simulink model "VIENNA_"  (R2021a)
settings: Solver=ode45  StartTime=0.0  StopTime=0.45  RelTol=1e-3  EnableMultiTasking=on
libraries: spsDiodeLib x6, spsMosfetLib x6, spsSeriesRLCBranchLib x6, spsVoltageMeasurementLib x3, spsCurrentMeasurementLib x1, spsDCMachineLib x1, spsDCVoltageSourceLib x1, spsMeanLib x1, spsPower3phInstantaneousLib x1, slpidlib x1, spsThreePhaseVIMeasurementLib x1, spsThreePhaseSourceLib x1
settings Model: Creator=Zhaoxuqiang  LastModifiedBy=Saghana
settings SolverCC: AlgebraicLoopSolver=TrustRegion
settings DataIOCC: LimitDataPoints=on  SaveFormat=Array  ReturnWorkspaceOutputs=off
settings OptimizationCC: LifeSpan=inf
settings DebuggingCC: SolverPrmCheckMsg=warning  SFUnexpectedBacktrackingDiag=warning  SFNoUnconditionalDefaultTransitionDiag=warning  SFExecutionAtInitializationDiag=none  SFMachineParentedDataDiag=warning  ArithmeticOperatorsInVariantConditions=warning
settings HardwareCC: ProdBitPerPointer=32  ProdBitPerSizeT=32  ProdBitPerPtrDiffT=32  ProdLargestAtomicFloat=None  ProdIntDivRoundTo=Undefined  ProdEndianess=Unspecified  ProdWordSize=32  ProdHWDeviceType=32-bit Generic
settings ModelReferenceCC: PropagateSignalLabelsOutOfModel=off
settings SFSimCC: SimUseLocalCustomCode=off  CustomCodeUndefinedFunction=UseInterfaceOnly
settings RTWCC: RTWUseLocalCustomCode=off
settings CodeAppCC: StateflowObjectComments=on
settings GRTTargetCC: TargetLangStandard=C89/C90 (ANSI)
settings ConfigComp: CovMetricSettings=dw  CovSaveCumulativeToWorkspaceVar=on  CovSaveSingleToWorkspaceVar=on  CovExternalEMLEnable=off  CovSFcnEnable=off
settings SimscapeCC: SimscapeNormalizeSystem=off

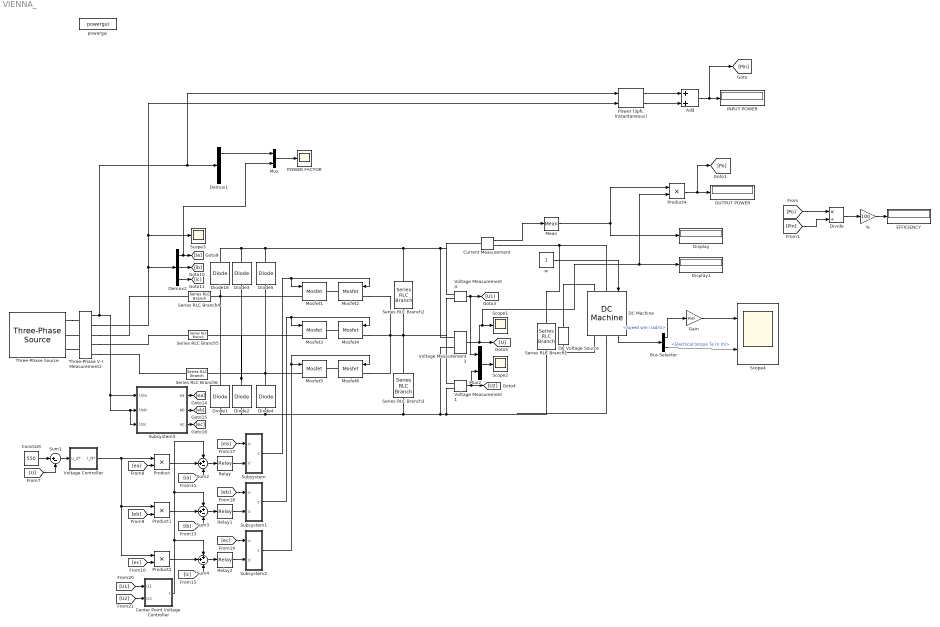
== system VIENNA_ ==
  % : Gain  Gain=100
  Add : Sum
  Bus Selector : BusSelector  OutputSignals=Speed wm (rad/s),Electrical torque Te (n m)
  Center Point Voltage Controller : Subsystem
  Constant : Constant  Value=550
  Current Measurement : spsCurrentMeasurementLib/Current Measurement  PhasorSimulation=off  OutputType=Complex  PSBequivalent=0
  DC Machine : spsDCMachineLib/DC Machine  PresetModel=03: 5HP 500V 1750RPM Field:300V  MechanicalLoad=Torque TL  FieldType=Wound  ShowDetailedParameters=on  MeasurementBus=off  RLa=[11.2 0.1215]  RLf=[281.2 156]  Laf=1.976  MachineConstant=Torque constant (N.m/A)  Ke=1.8  Kt=1.8  J=0.02215  Bm=0.002953  Tf=0.5161  w0=1  Ifinit=1.06685632871799  TsPowergui=0  TsBlock=-1
  DC Voltage Source : spsDCVoltageSourceLib/DC Voltage Source  Amplitude=300  Measurements=None
  Demux1 : Demux  Outputs=3
  Demux2 : Demux  Outputs=3
  Diode{1..5,18} (6 alike) : spsDiodeLib/Diode  Ron=0.001  Lon=0  Vf=0.8  IC=0  UseSnubber=off  Rs=500  Cs=250e-9  Measurements=off
  Display : Display
  Display1 : Display
  Divide : Product  Inputs=*/
  EFFICIENCY : Display
  Gain : Gain  Gain=30/pi
  INPUT POWER : Display
  Mean : spsMeanLib/Mean  Freq=60  Vinit=0  Ts=0
  Mosfet{1..6} (6 alike) : spsMosfetLib/Mosfet  Ron=0.1  Lon=0  Rd=0.01  Vfd=0  IC=0  Rs=1e5  Cs=inf  Measurements=off
  Mux : Mux  Inputs=2
  Mux2 : Mux  Inputs=2
  OUTPUT POWER : Display
  POWER FACTOR : Scope
  "Power (3ph, Instantaneous)" : spsPower3phInstantaneousLib/Power (3ph, Instantaneous)
  Product : Product  RndMeth=Zero
  Product1 : Product  RndMeth=Zero
  Product2 : Product  RndMeth=Zero
  Product4 : Product
  Relay : Relay  OnSwitchValue=1  OffSwitchValue=-1
  Relay1 : Relay  OnSwitchValue=1  OffSwitchValue=-1
  Relay2 : Relay  OnSwitchValue=1  OffSwitchValue=-1
  Scope1 : Scope
  Scope2 : Scope
  Scope3 : Scope
  Scope4 : Scope  NumInputPorts=2
  Series RLC Branch1 : spsSeriesRLCBranchLib/Series RLC Branch  LConnTagsString=__new0  RConnTagsString=__new0  BranchType=R  Resistance=50  Inductance=1e-3  SetiL0=off  InitialCurrent=0  Capacitance=4000e-6  Setx0=on  InitialVoltage=200  Measurements=None
  Series RLC Branch2 : spsSeriesRLCBranchLib/Series RLC Branch  LConnTagsString=__new0  RConnTagsString=__new0  BranchType=C  Resistance=0.001  Inductance=1e-3  SetiL0=off  InitialCurrent=0  Capacitance=4000e-6  Setx0=on  InitialVoltage=200  Measurements=None
  Series RLC Branch3 : spsSeriesRLCBranchLib/Series RLC Branch  LConnTagsString=__new0  RConnTagsString=__new0  BranchType=C  Resistance=0.002  Inductance=1e-3  SetiL0=off  InitialCurrent=0  Capacitance=4000e-6  Setx0=on  InitialVoltage=400  Measurements=None
  Series RLC Branch4 : spsSeriesRLCBranchLib/Series RLC Branch  LConnTagsString=__new0  RConnTagsString=__new0  BranchType=L  Resistance=1  Inductance=0.3e-3  SetiL0=off  InitialCurrent=0  Capacitance=1e-6  Setx0=off  InitialVoltage=0  Measurements=None
  Series RLC Branch5 : spsSeriesRLCBranchLib/Series RLC Branch  LConnTagsString=__new0  RConnTagsString=__new0  BranchType=L  Resistance=1  Inductance=0.3e-3  SetiL0=off  InitialCurrent=0  Capacitance=1e-6  Setx0=off  InitialVoltage=0  Measurements=None
  Series RLC Branch6 : spsSeriesRLCBranchLib/Series RLC Branch  LConnTagsString=__new0  RConnTagsString=__new0  BranchType=L  Resistance=1  Inductance=0.3e-3  SetiL0=off  InitialCurrent=0  Capacitance=1e-6  Setx0=off  InitialVoltage=0  Measurements=None
  Subsystem : Subsystem
  Subsystem1 : Subsystem
  Subsystem2 : Subsystem
  Subsystem3 : Subsystem
      mask Display: disp('PLL');
  Sum1 : Sum  Inputs=|+-
  Sum2 : Sum  Inputs=++-
  Sum3 : Sum  Inputs=++-
  Sum4 : Sum  Inputs=++-
  Three-Phase V-I Measurement2 : spsThreePhaseVIMeasurementLib/Three-Phase V-I Measurement  VoltageMeasurement=phase-to-ground  SetLabelV=off  LabelV=Uabc  Vpu=off  VpuLL=off  CurrentMeasurement=yes  SetLabelI=off  LabelI=Iabc  Ipu=off  Pbase=100e6  Vbase=500e3  OutputType=Complex  PhasorSimulation=off  PSBequivalent=0
  Three-Phase Source : spsThreePhaseSourceLib/Three-Phase Source  InternalConnection=Yg  VoltagePhases=off  Voltage=380  PhaseAngle=0  Voltage_phases=[25e3 25e3 25e3]/sqrt(3)  PhaseAngles_phases=[0 -120 +120]  Frequency=50  NonIdealSource=on  SpecifyImpedance=off  Resistance=0.000001  Inductance=0  ShortCircuitLevel=100e6  BaseVoltage=25e3  XRratio=7  BusType=swing  Pref=0  Qref=0  Prefabc=[10e3, 10e3, 10e3]  Qrefabc=[0, 0, 0]  Qmin=-inf  Qmax=inf
  Voltage Controller : Subsystem
      mask Display: disp('PI');
  Voltage Measurement1 : spsVoltageMeasurementLib/Voltage Measurement  PhasorSimulation=off  OutputType=Complex  PSBequivalent=0
  Voltage Measurement3 : spsVoltageMeasurementLib/Voltage Measurement  PhasorSimulation=off  OutputType=Complex  PSBequivalent=0
  Voltage Measurement4 : spsVoltageMeasurementLib/Voltage Measurement  PhasorSimulation=off  OutputType=Complex  PSBequivalent=0
  powergui : spspowerguiLib/powergui  SimulationMode=Continuous  SampleTime=1e-6  frequency=60  Iterations=50  frequencyindice=50  Pbase=100e6  ErrMax=1e-4  UnitsV=kV  UnitsW=MW  buscounter=0  FunctionMessages=off  echomessages=off  EnableUseOfTLC=off  CurrentSourceSwitches=on  DisableSnubberDevices=off  DisableRonSwitches=off  DisableVfSwitches=off  DisplayEquations=off  AutomaticDiscreteSolvers=off  SolverType=Tustin/Backward Euler (TBE)  Interpol=off  ExternalGateDelay=off  methode=off  Ts=0  x0status=blocks  SPID=off  SwTol=0  HookPort=off  NonlinearTolerance=1e-4  nMaxIteration=100  ContinueOnMaxIteration=off  RestoreLinks=warning  ResistiveCurrentMeasurement=off  Frange=[0:2:500]  Ylog=off  Xlog=on  ShowGrid=off  save=off  variable=ZData  structure=Iabc  ZoomFFT=off  StartTime=0.3  cycles=10  DisplayStyle=1  fundamental=50  FreqAxis=on  MaxFrequency=2500  frequencyindicesteady=1  RmsSteady=1  display=off
  w : Constant
  wires:
  Voltage Measurement3/1 -> Product4/2, Display1/1, Scope1/1, [U]
  Voltage Measurement1/1 -> Mux2/2, [U2]
  Voltage Measurement4/1 -> Mux2/1, [U1]
  Constant/1 -> Sum1/1
  Sum1/1 -> Voltage Controller/1(u_d*)
  [U] -> Sum1/2
  [ea] -> Product/2
  [eb] -> Product1/2
  Voltage Controller/1(I_N*) -> Product2/1, Product1/1, Product/1
  [ec] -> Product2/2
  Product/1 -> Sum2/2
  Demux2/2 -> [ib]
  Demux2/1 -> Mux/2, [ia]
  Demux2/3 -> [ic]
  [ia] -> Sum2/3
  Product1/1 -> Sum3/2
  [ib] -> Sum3/3
  Product2/1 -> Sum4/2
  [ic] -> Sum4/3
  Center Point Voltage Controller/1(I) -> Sum4/1, Sum3/1, Sum2/1
  Relay/1 -> Subsystem/2(s')
  [ea] -> Subsystem/1(u)
  Sum2/1 -> Relay/1
  Relay1/1 -> Subsystem1/2(s')
  [eb] -> Subsystem1/1(u)
  Sum3/1 -> Relay1/1
  Relay2/1 -> Subsystem2/2(s')
  [ec] -> Subsystem2/1(u)
  Sum4/1 -> Relay2/1
  [U1] -> Center Point Voltage Controller/1(U1)
  [U2] -> Center Point Voltage Controller/2(U2)
  Subsystem/1(s) -> Mosfet2/1, Mosfet1/1
  Subsystem1/1(s) -> Mosfet4/1, Mosfet3/1
  Subsystem2/1(s) -> Mosfet5/1, Mosfet6/1
  Three-Phase V-I Measurement2/1 -> "Power (3ph, Instantaneous)"/1, Demux1/1, Subsystem3/1(Uoa), Subsystem3/3(Uoc), Subsystem3/2(Uob)
  Subsystem3/1(ea) -> [ea]
  Subsystem3/2(eb) -> [eb]
  Subsystem3/3(ec) -> [ec]
  Mux2/1 -> Scope2/1
  w/1 -> DC Machine/1
  DC Machine/1 -> Bus Selector/1
  Bus Selector/1 -> Gain/1  "<Speed wm (rad/s)>"
  Bus Selector/2 -> Scope4/2  "<Electrical torque Te (n m)>"
  Mux/1 -> POWER FACTOR/1
  Current Measurement/1 -> Mean/1
  Demux1/1 -> Mux/1
  Gain/1 -> Scope4/1
  Product4/1 -> [Po], OUTPUT POWER/1
  "Power (3ph, Instantaneous)"/1 -> Add/1
  "Power (3ph, Instantaneous)"/2 -> Add/2
  Add/1 -> INPUT POWER/1, [Pin]
  [Po] -> Divide/1
  [Pin] -> Divide/2
  Divide/1 -> %/1
  %/1 -> EFFICIENCY/1
  Mean/1 -> Display/1, Product4/1
  Three-Phase V-I Measurement2/2 -> "Power (3ph, Instantaneous)"/2, Scope3/1, Demux2/1
  connections:
  Three-Phase V-I Measurement2/RConn3 -- Series RLC Branch6/LConn1
  Three-Phase V-I Measurement2/RConn2 -- Series RLC Branch5/LConn1
  Three-Phase V-I Measurement2/RConn1 -- Series RLC Branch4/LConn1
  Three-Phase V-I Measurement2/LConn3 -- Three-Phase Source/RConn3
  Three-Phase Source/RConn1 -- Three-Phase V-I Measurement2/LConn1
  Three-Phase V-I Measurement2/LConn2 -- Three-Phase Source/RConn2
  Mosfet4/LConn1 -- Mosfet6/LConn1 -- Voltage Measurement1/LConn1 -- Voltage Measurement4/LConn2 -- Series RLC Branch3/LConn1 -- Series RLC Branch2/RConn1 -- Mosfet2/LConn1
  Diode3/RConn1 -- Diode18/RConn1 -- Voltage Measurement4/LConn1 -- Current Measurement/LConn1 -- Voltage Measurement3/LConn1 -- Series RLC Branch2/LConn1 -- Diode5/RConn1
  Diode4/LConn1 -- Voltage Measurement3/LConn2 -- DC Machine/RConn1 -- Series RLC Branch1/RConn1 -- Voltage Measurement1/LConn2 -- Series RLC Branch3/RConn1 -- Diode1/LConn1 -- Diode2/LConn1
  Mosfet5/LConn1 -- Diode5/LConn1 -- Series RLC Branch6/RConn1 -- Diode4/RConn1
  Diode2/RConn1 -- Diode3/LConn1 -- Series RLC Branch5/RConn1 -- Mosfet3/LConn1
  Diode1/RConn1 -- Series RLC Branch4/RConn1 -- Mosfet1/LConn1 -- Diode18/LConn1
  Mosfet2/RConn1 -- Mosfet1/RConn1
  Mosfet4/RConn1 -- Mosfet3/RConn1
  Mosfet6/RConn1 -- Mosfet5/RConn1
  DC Voltage Source/RConn1 -- DC Machine/LConn2
  DC Machine/RConn2 -- DC Voltage Source/LConn1
  Current Measurement/RConn1 -- Series RLC Branch1/LConn1 -- DC Machine/LConn1

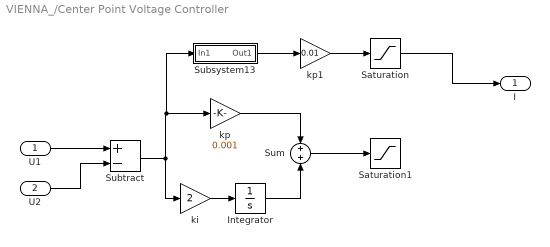
== system VIENNA_/Center Point Voltage Controller ==
  U1 : Inport
  U2 : Inport  Port=2
  Integrator : Integrator  LimitOutput=on  UpperSaturationLimit=0.5  LowerSaturationLimit=-0.5
  Saturation : Saturate
  Saturation1 : Saturate
  Subsystem13 : Subsystem
      mask Display: disp('LPF')
  Subtract : Sum  Inputs=+-
  Sum : Sum  Inputs=+|+
  ki : Gain  Gain=2
  kp : Gain  Gain=0.001
  kp1 : Gain  Gain=0.01
  I : Outport
  wires:
  U1/1 -> Subtract/1
  U2/1 -> Subtract/2
  Subtract/1 -> ki/1, Subsystem13/1(In1), kp/1
  ki/1 -> Integrator/1
  kp/1 -> Sum/1
  Integrator/1 -> Sum/2
  Subsystem13/1(Out1) -> kp1/1
  kp1/1 -> Saturation/1
  Sum/1 -> Saturation1/1
  Saturation/1 -> I/1

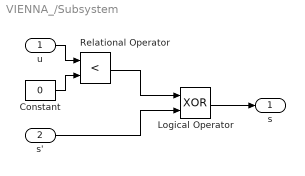
== system VIENNA_/Subsystem ==
  u : Inport
  s' : Inport  Port=2
  Constant : Constant  Value=0
  Logical Operator : Logic  Operator=XOR  AllPortsSameDT=off  OutDataTypeStr=boolean
  Relational Operator : RelationalOperator  Operator=<  OutDataTypeStr=boolean  RndMeth=Nearest
  s : Outport
  wires:
  Logical Operator/1 -> s/1
  u/1 -> Relational Operator/1
  Constant/1 -> Relational Operator/2
  Relational Operator/1 -> Logical Operator/1
  s'/1 -> Logical Operator/2

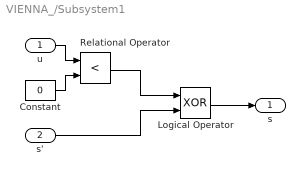
== system VIENNA_/Subsystem1 ==
  u : Inport
  s' : Inport  Port=2
  Constant : Constant  Value=0
  Logical Operator : Logic  Operator=XOR  AllPortsSameDT=off  OutDataTypeStr=boolean
  Relational Operator : RelationalOperator  Operator=<  OutDataTypeStr=boolean  RndMeth=Nearest
  s : Outport
  wires:
  s'/1 -> Logical Operator/2
  Relational Operator/1 -> Logical Operator/1
  Constant/1 -> Relational Operator/2
  u/1 -> Relational Operator/1
  Logical Operator/1 -> s/1

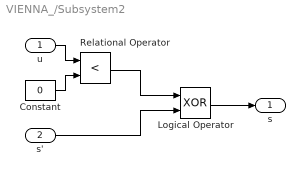
== system VIENNA_/Subsystem2 ==
  u : Inport
  s' : Inport  Port=2
  Constant : Constant  Value=0
  Logical Operator : Logic  Operator=XOR  AllPortsSameDT=off  OutDataTypeStr=boolean
  Relational Operator : RelationalOperator  Operator=<  OutDataTypeStr=boolean  RndMeth=Nearest
  s : Outport
  wires:
  Logical Operator/1 -> s/1
  u/1 -> Relational Operator/1
  Constant/1 -> Relational Operator/2
  Relational Operator/1 -> Logical Operator/1
  s'/1 -> Logical Operator/2

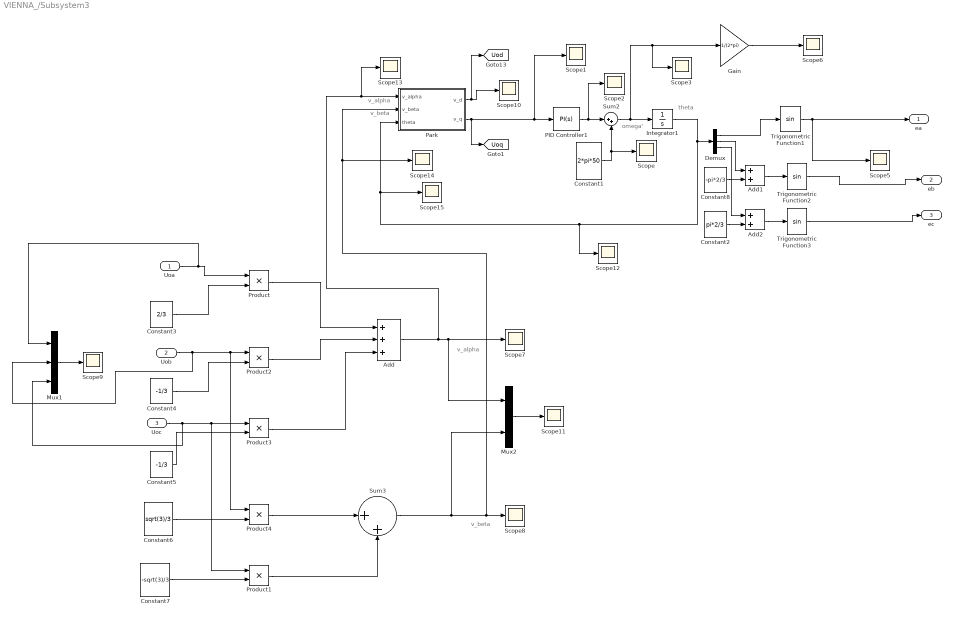
== system VIENNA_/Subsystem3 ==
  note: v_alpha
  note: v_beta
  note: v_beta
  note: v_alpha
  note: theta
  note: omega'
  Uoa : Inport
  Uob : Inport  Port=2
  Uoc : Inport  Port=3
  Add : Sum  Inputs=+++
  Add1 : Sum
  Add2 : Sum
  Constant1 : Constant  Value=2*pi*50
  Constant2 : Constant  Value=pi*2/3
  Constant3 : Constant  Value=2/3
  Constant4 : Constant  Value=-1/3
  Constant5 : Constant  Value=-1/3
  Constant6 : Constant  Value=sqrt(3)/3
  Constant7 : Constant  Value=-sqrt(3)/3
  Constant8 : Constant  Value=-pi*2/3
  Demux : Demux  Outputs=3
  Gain : Gain  Gain=1/(2*pi)
  Integrator1 : Integrator
  Mux1 : Mux  Inputs=3
  Mux2 : Mux  Inputs=2
  PID Controller1 : slpidlib/PID Controller  Controller=PI  Form=Parallel  TimeDomain=Continuous-time  UseExternalTs=off  SampleTime=-1  IntegratorMethod=Forward Euler  FilterMethod=Forward Euler  ControllerParametersSource=internal  P=184  I=16928  D=0  UseFilter=on  N=100  TunerSelectOption=Transfer Function Based (PID Tuner App)  InitialConditionSource=internal  InitialConditionForIntegrator=0  InitialConditionForFilter=0  DifferentiatorICPrevScaledInput=0  ExternalReset=none  TrackingMode=off  Kt=1  LimitOutput=off  SatLimitsSource=internal  UpperSaturationLimit=inf  LowerSaturationLimit=-inf  LinearizeAsGain=off  AntiWindupMode=none  Kb=1  POutMin=[]  POutMax=[]  IOutMin=[]  IOutMax=[]  DOutMin=[]  DOutMax=[]  NOutMin=[]  NOutMax=[]  SumOutMin=[]  SumOutMax=[]  SaturationOutMin=[]  SaturationOutMax=[]  PParamMin=[]  PParamMax=[]  IParamMin=[]  IParamMax=[]  DParamMin=[]  DParamMax=[]  NParamMin=[]  NParamMax=[]  KbParamMin=[]  KbParamMax=[]  KtParamMin=[]  KtParamMax=[]  KbOutMin=[]  KbOutMax=[]  KtOutMin=[]  KtOutMax=[]  IntegratorOutMin=[]  IntegratorOutMax=[]  FilterOutMin=[]  FilterOutMax=[]  SumI1OutMin=[]  SumI1OutMax=[]  SumI2OutMin=[]  SumI2OutMax=[]  SumI3OutMin=[]  SumI3OutMax=[]  SumI4OutMin=[]  SumI4OutMax=[]  SumDOutMin=[]  SumDOutMax=[]  DifferentiatorOutMin=[]  DifferentiatorOutMax=[]  FilterDiffOutCoefMin=[]  FilterDiffOutCoefMax=[]  ReciprocalOutMin=[]  ReciprocalOutMax=[]  SumDenOutMin=[]  SumDenOutMax=[]  SumNumOutMin=[]  SumNumOutMax=[]  DivideOutMin=[]  DivideOutMax=[]  UdiffTsProdOutMin=[]  UdiffTsProdOutMax=[]  NTsProdOutMin=[]  NTsProdOutMax=[]  UintegralTsProdOutMin=[]  UintegralTsProdOutMax=[]  UngainTsProdOutMin=[]  UngainTsProdOutMax=[]  IntegratorContinuousStateAttributes=''  IntegratorStateMustResolveToSignalObject=off  IntegratorRTWStateStorageClass=Auto  FilterContinuousStateAttributes=''  FilterStateMustResolveToSignalObject=off  FilterRTWStateStorageClass=Auto  ParallelPVariant=InternalParameters  IdealPVariant=Disabled  IVariant=InternalParameters  DVariant=Disabled  IntegratorVariant=Continuous  SatVariant=Disabled  AWVariant=Passthrough  PCopyVariant=Disabled  TRVariant=Disabled  FdbkBlocksVariant=Forward  IdealPFdbkVariant=Disabled  SatFdbkVariant=Disabled  DerivativeFilterVariant=Disabled  NVariant=Disabled  NCopyVariant=Disabled_SignalSpec  FilterICVariant=Disabled  IntegratorICVariant=InternalICs  ExternalResetVariant=Disabled  TRSumVariant=Passthrough  SumFdbkVariant=Disabled  SumVariant=Sum_PI  TsampFilterVariant=InternalTs  TsampNgainVariant=Passthrough  TsampIntegralVariant=Passthrough  ExternalSaturationOutDataTypeStr=Inherit: Same as second input
  Park : Subsystem
      mask Display: disp('   Park');
  Product{,1..4} (5 alike) : Product  RndMeth=Zero
  Scope{,1..3,5..15} (15 alike) : Scope
  Sum2 : Sum  Inputs=|++
  Sum3 : Sum  Inputs=|++
  Trigonometric Function1 : Trigonometry
  Trigonometric Function2 : Trigonometry
  Trigonometric Function3 : Trigonometry
  ea : Outport
  eb : Outport  Port=2
  ec : Outport  Port=3
  tag scope: Uod=global, Uoq=global
  wires:
  Park/2(v_q) -> [Uoq], PID Controller1/1, Scope1/1
  PID Controller1/1 -> Sum2/1, Scope2/1
  Constant1/1 -> Sum2/2, Scope/1
  Sum2/1 -> Integrator1/1, Gain/1, Scope3/1
  Trigonometric Function1/1 -> ea/1, Scope5/1
  Gain/1 -> Scope6/1
  Uoa/1 -> Product/1, Mux1/1
  Constant3/1 -> Product/2
  Uob/1 -> Product2/1, Product4/1, Mux1/2
  Constant4/1 -> Product2/2
  Constant5/1 -> Product3/2
  Product/1 -> Add/1
  Product2/1 -> Add/2
  Product3/1 -> Add/3
  Constant6/1 -> Product4/2
  Constant7/1 -> Product1/2
  Product4/1 -> Sum3/1
  Product1/1 -> Sum3/2
  Add/1 -> Scope7/1, Mux2/1, Park/1(v_alpha), Scope13/1
  Sum3/1 -> Mux2/2, Scope8/1, Park/2(v_beta), Scope14/1
  Mux1/1 -> Scope9/1
  Mux2/1 -> Scope11/1
  Uoc/1 -> Product3/1, Product1/1, Mux1/3
  Park/1(v_d) -> [Uod], Scope10/1
  Trigonometric Function2/1 -> eb/1
  Trigonometric Function3/1 -> ec/1
  Add1/1 -> Trigonometric Function2/1
  Add2/1 -> Trigonometric Function3/1
  Constant8/1 -> Add1/2
  Integrator1/1 -> Scope12/1, Park/3(theta), Scope15/1, Demux/1
  Constant2/1 -> Add2/2
  Demux/1 -> Trigonometric Function1/1
  Demux/2 -> Add1/1
  Demux/3 -> Add2/1

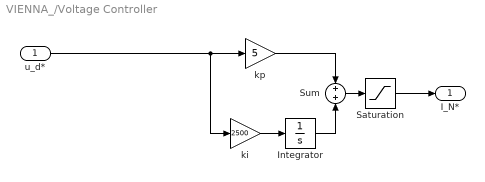
== system VIENNA_/Voltage Controller ==
  u_d* : Inport
  Integrator : Integrator  LimitOutput=on  UpperSaturationLimit=150  LowerSaturationLimit=0
  Saturation : Saturate  UpperLimit=150  LowerLimit=0
  Sum : Sum  Inputs=+|+
  ki : Gain  Gain=2500
  kp : Gain  Gain=5
  I_N* : Outport
  wires:
  Sum/1 -> Saturation/1
  kp/1 -> Sum/1
  Integrator/1 -> Sum/2
  ki/1 -> Integrator/1
  u_d*/1 -> ki/1, kp/1
  Saturation/1 -> I_N*/1

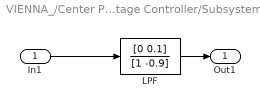
== system VIENNA_/Center Point Voltage Controller/Subsystem13 ==
  In1 : Inport
  LPF : DiscreteFilter  Numerator=[0 0.1]  Denominator=[1 -0.9]  SampleTime=1e-3
  Out1 : Outport
  wires:
  In1/1 -> LPF/1
  LPF/1 -> Out1/1

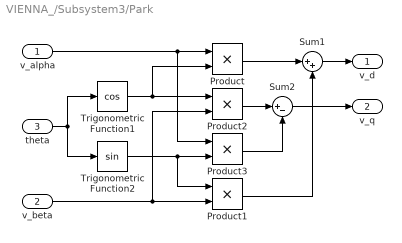
== system VIENNA_/Subsystem3/Park ==
  v_alpha : Inport
  v_beta : Inport  Port=2
  theta : Inport  Port=3
  Product{,1..3} (4 alike) : Product  RndMeth=Zero
  Sum1 : Sum  Inputs=|++
  Sum2 : Sum  Inputs=|+-
  Trigonometric Function1 : Trigonometry  Operator=cos
  Trigonometric Function2 : Trigonometry
  v_d : Outport
  v_q : Outport  Port=2
  wires:
  v_beta/1 -> Product1/2, Product2/2
  v_alpha/1 -> Product/1, Product3/1
  Product/1 -> Sum1/1
  Product1/1 -> Sum1/2
  Product2/1 -> Sum2/1
  Product3/1 -> Sum2/2
  Sum1/1 -> v_d/1
  Sum2/1 -> v_q/1
  Trigonometric Function2/1 -> Product3/2, Product1/1
  theta/1 -> Trigonometric Function1/1, Trigonometric Function2/1
  Trigonometric Function1/1 -> Product2/1, Product/2
